simulink subsystem "Car"  (R2022b)
settings: Solver=VariableStepAuto  StartTime=0.0  StopTime=10.0  RelTol=1e-3
model mask{InitPos=0, InitVol=0}
  mask prompts: InitPos "Initial position (m)"; InitVol "Initial velocity (Km/hr)"
settings Model: Creator=MAAM  LastModifiedBy=MAAM

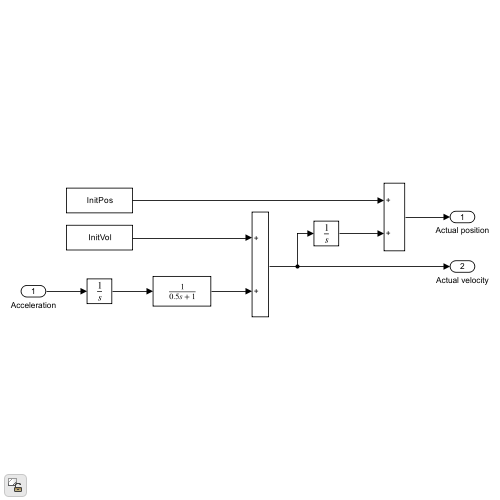
[thumbnail: Simulink's stored preview of the top-level diagram]
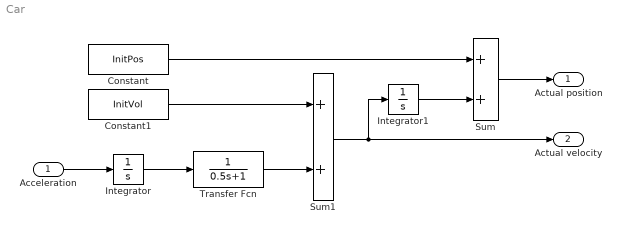
== system Car ==
  Acceleration : Inport
  Constant : Constant  Value=InitPos  OutDataTypeStr=Inherit: Inherit via back propagation
  Constant1 : Constant  Value=InitVol  OutDataTypeStr=Inherit: Inherit via back propagation
  Integrator : Integrator
  Integrator1 : Integrator
  Sum : Sum  OutDataTypeStr=Inherit: Inherit via back propagation
  Sum1 : Sum  OutDataTypeStr=Inherit: Inherit via back propagation
  Transfer Fcn : TransferFcn  Denominator=[0.5 1]
  Actual position : Outport  VectorParamsAs1DForOutWhenUnconnected=off
  Actual velocity : Outport  Port=2  VectorParamsAs1DForOutWhenUnconnected=off
  wires:
  Integrator1/1 -> Sum/2
  Constant/1 -> Sum/1
  Acceleration/1 -> Integrator/1
  Sum1/1 -> Integrator1/1, Actual velocity/1
  Integrator/1 -> Transfer Fcn/1
  Sum/1 -> Actual position/1
  Constant1/1 -> Sum1/1
  Transfer Fcn/1 -> Sum1/2
